simulink model "etc_reg"  (Simulink 5.0)
settings: Solver=ode15s  StartTime=0.0  StopTime=0.2  FixedStep=1e-3  RelTol=1e-5  AbsTol=1e-10
PreLoadFcn:
  | setup_reg
libraries: cmlib x6, simulink x1
settings Model: LastModifiedBy=ansgar  ExtModeTrigMode=oneshot  ExtModeArmWhenConnect=off  LimitDataPoints=off  BlockReductionOpt=off

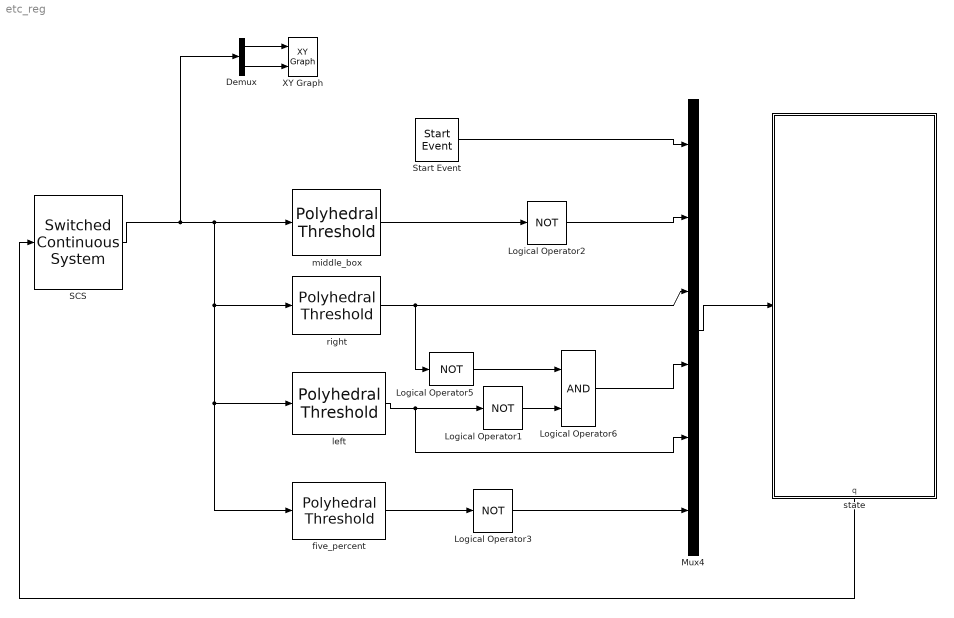
== system etc_reg ==
  Demux : Demux  Outputs=2
  Logical Operator{1..3,5} (4 alike) : Logic  Operator=NOT
  Logical Operator6 : Logic
  Mux4 : Mux  Inputs=6
  SCS : cmlib/Switched Continuous System  AncestorBlock=cmlib/Switched Continuous System  nx=2  use_sd=off  nup=[]  nz=[]  use_reset=off  nu=1  x0=[1.606488;-0.22]  swfunc=slidingmode_reg  ICS=etc_ICS  AR=etc_AR  use_param=on  p0=[1;1]  PaCs=etc_PaCs
  Start Event : cmlib/Start Event  steptime=0.0001  initval=0  finival=1  sampletime=0  interpret=on  enable=on
  XY Graph : simulink/Sinks/XY Graph  xmin=1.59  xmax=1.61  ymin=-2.5  ymax=0  st=-1
  five_percent : cmlib/Polyhedral Threshold  polyhedron=five_percent
  left : cmlib/Polyhedral Threshold  polyhedron=turn_left
  middle_box : cmlib/Polyhedral Threshold  polyhedron=above_surf
  right : cmlib/Polyhedral Threshold  polyhedron=turn_right
  state : Stateflow chart  Orientation=down  TreatAsAtomicUnit=on
  wires:
  Mux4/1 -> state/Trigger
  SCS/1 -> middle_box/1, right/1, left/1, five_percent/1, Demux/1
  left/1 -> Logical Operator1/1, Mux4/5
  state/1(q) -> SCS/1
  right/1 -> Logical Operator5/1, Mux4/3
  Start Event/1 -> Mux4/1
  Logical Operator1/1 -> Logical Operator6/2
  Logical Operator5/1 -> Logical Operator6/1
  middle_box/1 -> Logical Operator2/1
  Logical Operator6/1 -> Mux4/4
  Logical Operator2/1 -> Mux4/2
  five_percent/1 -> Logical Operator3/1
  Logical Operator3/1 -> Mux4/6
  Demux/1 -> XY Graph/1
  Demux/2 -> XY Graph/2

== stateflow chart state ==
  state left
    entry: q=1;
  state right
    entry: q=3;
  state neither
    entry: q=2;
  state reach
    entry: q=4;
  state avoid
    entry: q=5;
  left -> neither : negturn
  (default) -> left : start
  right -> neither : negturn
  neither -> right : turnright
  neither -> left : turnleft
  left -> reach : middle_box
  neither -> reach : middle_box
  right -> reach : middle_box
  left -> avoid : out_spec
  neither -> avoid : out_spec
  right -> avoid : out_spec
  data: q output int16
  events: start input RISING_EDGE_EVENT; middle_box input RISING_EDGE_EVENT; turnleft input RISING_EDGE_EVENT; negturn input RISING_EDGE_EVENT; turnright input RISING_EDGE_EVENT; out_spec input RISING_EDGE_EVENT
